simulink model "Practica1_DAMR"  (R2024a)
settings: Solver=VariableStepAuto  StartTime=0.0  StopTime=10.0  RelTol=1e-3
InitFcn:
  | m1=0.2;
  | l1=0.3;
  | m2=0.1;
  | l2=0.25;
  | g=9.81;
settings Model: Creator=Manuel  LastModifiedBy=Manuel

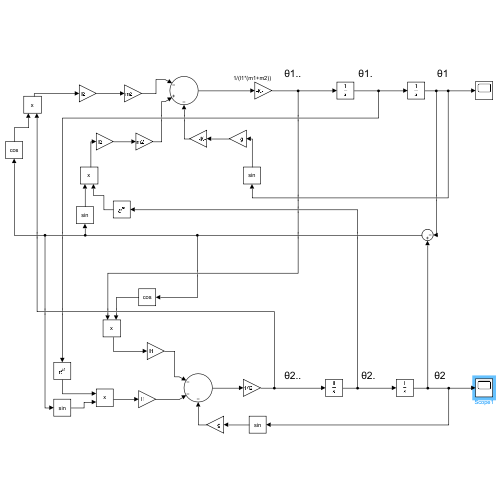
[thumbnail: Simulink's stored preview of the top-level diagram]
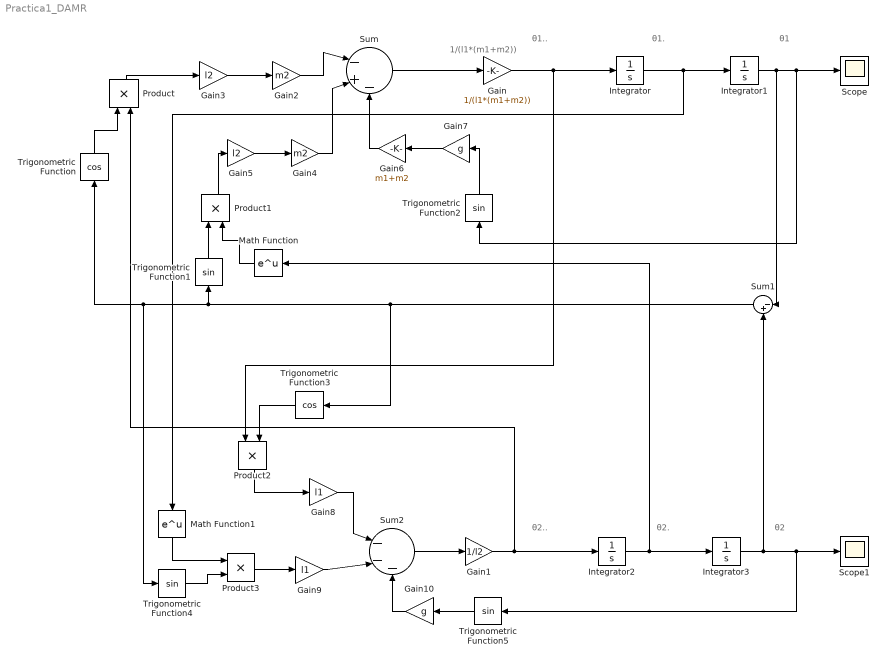
== system Practica1_DAMR ==
  note: θ2..
  note: θ2.
  note: θ2
  note: θ1..
  note: θ1.
  note: θ1
  note: 1/(l1*(m1+m2))
  Gain : Gain  Gain=1/(l1*(m1+m2))
  Gain1 : Gain  Gain=1/l2
  Gain10 : Gain  Gain=g
  Gain2 : Gain  Gain=m2
  Gain3 : Gain  Gain=l2
  Gain4 : Gain  Gain=m2
  Gain5 : Gain  Gain=l2
  Gain6 : Gain  Gain=m1+m2
  Gain7 : Gain  Gain=g
  Gain8 : Gain  Gain=l1
  Gain9 : Gain  Gain=l1
  Integrator : Integrator
  Integrator1 : Integrator
  Integrator2 : Integrator
  Integrator3 : Integrator  InitialCondition=35*(pi/180)
  Math Function : Math
  Math Function1 : Math
  Product{,1..3} (4 alike) : Product
  Scope : Scope
  Scope1 : Scope
  Sum : Sum  Inputs=|-+-
  Sum1 : Sum  Inputs=|-+
  Sum2 : Sum  Inputs=|---
  Trigonometric Function : Trigonometry  Operator=cos
  Trigonometric Function{1..2,4..5} (4 alike) : Trigonometry
  Trigonometric Function3 : Trigonometry  Operator=cos
  wires:
  Integrator/1 -> Math Function1/1, Integrator1/1
  Integrator3/1 -> Trigonometric Function5/1, Scope1/1, Sum1/2
  Gain1/1 -> Product/2, Integrator2/1
  Gain/1 -> Product2/1, Integrator/1
  Sum/1 -> Gain/1
  Gain2/1 -> Sum/1
  Gain3/1 -> Gain2/1
  Product/1 -> Gain3/1
  Trigonometric Function/1 -> Product/1
  Sum1/1 -> Trigonometric Function3/1, Trigonometric Function1/1, Trigonometric Function4/1, Trigonometric Function/1
  Gain5/1 -> Gain4/1
  Gain4/1 -> Sum/2
  Trigonometric Function1/1 -> Product1/1
  Integrator2/1 -> Math Function/1, Integrator3/1
  Math Function/1 -> Product1/2
  Product1/1 -> Gain5/1
  Integrator1/1 -> Sum1/1, Trigonometric Function2/1, Scope/1
  Trigonometric Function2/1 -> Gain7/1
  Gain7/1 -> Gain6/1
  Gain6/1 -> Sum/3
  Sum2/1 -> Gain1/1
  Product2/1 -> Gain8/1
  Trigonometric Function3/1 -> Product2/2
  Gain8/1 -> Sum2/1
  Gain9/1 -> Sum2/2
  Math Function1/1 -> Product3/1
  Trigonometric Function4/1 -> Product3/2
  Trigonometric Function5/1 -> Gain10/1
  Gain10/1 -> Sum2/3
  Product3/1 -> Gain9/1
